simulink library "ddm"  (R2021b)
settings: Solver=VariableStepAuto  StartTime=0.0  StopTime=10.0  RelTol=1e-3
undefined symbols (not defined in the file): ADDM_FrTMTqDev_X_Nm, ADDM_RrTMTqDev_X_Nm, ENUM_ADASACCSTA_ERROR, ENUM_ADASACCSTA_OFF, ENUM_ADASACCSTA_STANDBY, ENUM_ALLOWMOV_ALLOWREADY, ENUM_APS, ENUM_BRKSTA_ERROR, ENUM_BRKSTA_OFF, ENUM_BRKSTA_ON, ENUM_BRKSW_INVALID, ENUM_BRKSW_OFF, ENUM_BRKSW_ON, ENUM_CHGPREACTERRSTA_OBCPRE, ENUM_DCDCFAULTSTA_ANYFAULTLV1, ENUM_DCDCFAULTSTA_ANYFAULTLV2, ENUM_DRIVETRAIN_AWD, ENUM_DRIVETRAIN_FWD, ENUM_DRIVETRAIN_RWD, ENUM_EDUDRTSTA_NORMAL, ENUM_EPBERROR_FAILED, ENUM_EPBSTA_APPLIED, ENUM_EPBSTA_RELEASED, ENUM_ESCAPSSta_APSUNAVAILABLE, ENUM_GEARACTUALPOSN_INVALID, ENUM_GEARACTUALPOSN_P, ENUM_HVBATTREADYPRE_READY, ENUM_HWRESETSTA_HWRESETING, ENUM_MCUWARN_LV0, ENUM_MCUWARN_LV1, ENUM_MCUWARN_LV2, ENUM_MCUWARN_LV3, ENUM_MCUWARN_NOERROR, ENUM_OBCFAULTSTA_ANYFAULT, ENUM_PAS_R2F2, ENUM_PDFAULT_BATTPDFAIL, ENUM_PDFAULT_DCDCDISABLE, ENUM_PDFAULT_MCUDISABLE, ENUM_PDFAULT_MCUDISCHRG, ENUM_POWERSTA_OFF, ENUM_POWERSTA_ON, ENUM_POWERSTA_READY, ENUM_POWERSTA_STANDBY, ENUM_PRESSINDI_LOW, ENUM_PUFAULT_BATTUPFAIL, ENUM_PUFAULT_DCDCENABLEFAIL, ENUM_PUFAULT_PRECHRGCHKFAIL, ENUM_PUFAULT_SAFETYCHKFAIL, ENUM_PWRSTASW_OFF, ENUM_PWRSTASW_OFFA, ENUM_PWRSTASW_OFFCHVCHRG, ENUM_PWRSTASW_OFFCLVCHRG, ENUM_PWRSTASW_ON, ENUM_PWRSTASW_ONHVCHRG, ENUM_PWRSTASW_READY, ENUM_PWRSTASW_STANDBY, ENUM_RAPSErrWarnSta_NORMAL, ENUM_RAPSErrWarnSta_RAPSERRLV1, ENUM_SHIFTCOMMAND_P, ENUM_SHIFTERERRSTA_PBUTTONFAILURE ... (+471)
libraries: hcu_lib x540, simulink x3
(part 17 of 26)

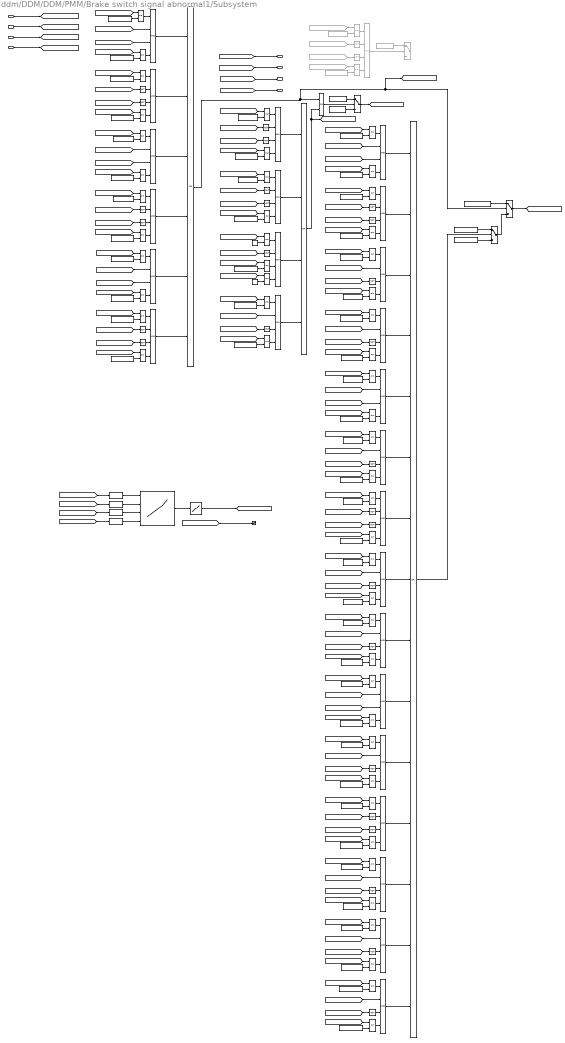
== system ddm/DDM/DDM/PMM/Brake switch signal abnormal1/Subsystem ==
  note: 17
  note: 6
  note: 35
  note: 25
  note: 27
  note: 30
  note: 12
  note: 19
  note: 3
  note: 21
  note: 1
  note: 9
  note: 11
  note: 36
  note: 24
  note: 33
  note: 29
  note: 13
  note: 5
  note: 23
  note: 18
  note: 15
  note: 20
  note: 24
  note: 17
  note: 3
  VDDM_CANBSW2S_enum : Inport
  BrakeSW : Inport  Port=2
  Brake_Stop_Lamp : Inport  Port=3
  BrkPedalPos_enum : Inport  Port=4
  1-D Lookup Table : Lookup_n-D  NumberOfTableDimensions=1  BreakpointsForDimension1=[1:36]  Table=[20,8,32,18,6,30,19,7,31,16,4,28,17,5,29,15,3,27,14,2,26,13,1,25,24,12,36,23,11,35,22,10,34,21,9,33]  ExtrapMethod=Clip  InternalRulePriority=Speed  RndMeth=Simplest  InputSameDT=on
  AND{,2..7,10,12..26,28..29} (25 alike) : Logic  Inputs=4  AllPortsSameDT=off  OutDataTypeStr=boolean
  AND1 : Logic  Operator=OR  Inputs=6  AllPortsSameDT=off  OutDataTypeStr=boolean
  AND11 : Logic  Operator=OR  Inputs=15  AllPortsSameDT=off  OutDataTypeStr=boolean
  AND27 : Logic  Commented=on  Inputs=4  AllPortsSameDT=off  OutDataTypeStr=boolean
  AND8 : Logic  Operator=OR  Inputs=4  AllPortsSameDT=off  OutDataTypeStr=boolean
  AND9 : Logic  Operator=OR  AllPortsSameDT=off  OutDataTypeStr=boolean
  Constant{1..10,15,17..18,23,29..30,32,49,52,54} (20 alike) : Constant  Value=ENUM_BRKSTA_ON
  Constant11 : Constant  Value=ENUM_BRKSW_OFF
  Constant{12..13,20,22,24,33..34,39,41..44,51} (13 alike) : Constant  Value=ENUM_BRKSTA_OFF
  Constant14 : Constant  Commented=on  Value=ENUM_BRKSTA_OFF
  Constant{16,19,21,25..28,31,38,50,53,55,57,59..61} (16 alike) : Constant  Value=ENUM_BRKSTA_ERROR
  Constant35 : Constant  Value=FALSE
  Constant36 : Constant  Value=TRUE
  Constant37 : Constant  Value=0
  Constant40 : Constant  Value=0
  Constant45 : Constant  Commented=on  Value=ENUM_BRKSTA_ERROR
  Constant46 : Constant  Value=ENUM_BRKSW_ON
  Constant47 : Constant  Value=ENUM_BRKSW_INVALID
  Constant48 : Constant  Commented=on  Value=FALSE
  Data Type Conversion{,1..3} (4 alike) : DataTypeConversion
  Equal{1..47,50..53} (51 alike) : RelationalOperator  Operator===  OutDataTypeStr=boolean  RndMeth=Simplest
  Equal48 : RelationalOperator  Commented=on  Operator===  OutDataTypeStr=boolean  RndMeth=Simplest
  Equal49 : RelationalOperator  Commented=on  Operator===  OutDataTypeStr=boolean  RndMeth=Simplest
  From100 : From  Commented=on  GotoTag=BrkPedalPos_enum
  From101 : From  Commented=on  GotoTag=BrakeSW
  From102 : From  Commented=on  GotoTag=VDDM_CANBSW2S_enum
  From103 : From  Commented=on  GotoTag=Brake_Stop_Lamp
  OR{,1..23,26..28} (27 alike) : Logic  Operator=NOT  AllPortsSameDT=off  OutDataTypeStr=boolean
  OR24 : Logic  Commented=on  Operator=NOT  AllPortsSameDT=off  OutDataTypeStr=boolean
  OR25 : Logic  Commented=on  Operator=NOT  AllPortsSameDT=off  OutDataTypeStr=boolean
  Switch1 : Switch  Commented=on  Criteria=u2 > Threshold
  Switch6 : Switch  Criteria=u2 > Threshold
  Switch7 : Switch  Criteria=u2 > Threshold
  Switch8 : Switch  Criteria=u2 > Threshold
  Terminator : Terminator
  n-D Lookup Table : Lookup_n-D  NumberOfTableDimensions=4  BreakpointsForDimension1=[0:2]  BreakpointsForDimension2=[0:1]  BreakpointsForDimension3=[0:1]  BreakpointsForDimension4=[0:2]  Table=reshape(1:36,[3,2,2,3])  ExtrapMethod=Clip  InternalRulePriority=Speed  RndMeth=Simplest  InputSameDT=on
      settings: InputPortMap=u0,u1,u2,u3
  BrkSWErr : Outport
  BrkSWNoBac : Outport  Port=2
  BrkSWPass : Outport  Port=3
  VDDM_BrakeSW_enum : Outport  Port=4
  wires:
  [VDDM_BrakeSigMatrix_enum] -> Terminator/1
  [VDDM_BrakeSW_enum] -> VDDM_BrakeSW_enum/1
  [BrkSWPass] -> BrkSWPass/1
  [BrkSWNoBac] -> BrkSWNoBac/1
  [BrkSWErr] -> BrkSWErr/1
  BrkPedalPos_enum/1 -> [BrkPedalPos_enum]
  Brake_Stop_Lamp/1 -> [Brake_Stop_Lamp]
  BrakeSW/1 -> [BrakeSW]
  VDDM_CANBSW2S_enum/1 -> [VDDM_CANBSW2S_enum]
  AND4/1 -> AND1/4
  Constant28/1 -> Equal14/2
  Constant31/1 -> Equal13/2
  Equal22/1 -> AND10/3
  Constant7/1 -> Equal3/2
  Equal33/1 -> AND19/4
  Equal39/1 -> AND22/4
  OR1/1 -> AND2/3
  [Brake_Stop_Lamp] -> OR8/1
  [Brake_Stop_Lamp] -> OR10/1
  Constant8/1 -> Equal8/2
  Equal17/1 -> AND7/1
  Constant50/1 -> Equal35/2
  Constant32/1 -> Equal41/2
  [BrkPedalPos_enum] -> Equal35/1
  Equal43/1 -> AND24/4
  Constant33/1 -> Equal26/2
  [VDDM_CANBSW2S_enum] -> Equal9/1
  Constant37/1 -> Equal20/2
  [BrkPedalPos_enum] -> Equal45/1
  Switch7/1 -> Switch8/3
  Equal36/1 -> AND21/1
  [Brake_Stop_Lamp] -> AND5/3
  Constant3/1 -> Equal17/2
  Constant44/1 -> Equal43/2
  Constant39/1 -> Equal30/2
  OR8/1 -> AND13/3
  [Brake_Stop_Lamp] -> OR19/1
  [VDDM_CANBSW2S_enum] -> Equal20/1
  Equal20/1 -> AND10/1
  [Brake_Stop_Lamp] -> Equal22/1
  [BrkPedalPos_enum] -> Equal6/1
  [VDDM_CANBSW2S_enum] -> Equal2/1
  Equal5/1 -> AND3/1
  [Brake_Stop_Lamp] -> OR3/1
  [Brake_Stop_Lamp] -> OR15/1
  Constant26/1 -> Equal11/2
  [Brake_Stop_Lamp] -> AND21/3
  OR19/1 -> AND24/3
  [BrkPedalPos_enum] -> Equal10/1
  [BrakeSW] -> AND25/2
  OR3/1 -> AND4/3
  Equal31/1 -> AND18/4
  [BrkPedalPos_enum] -> Equal31/1
  [VDDM_CANBSW2S_enum] -> Equal38/1
  Equal13/1 -> AND6/4
  AND9/1 -> Switch6/2
  [VDDM_CANBSW2S_enum] -> Equal17/1
  [Brake_Stop_Lamp] -> AND16/3
  Equal18/1 -> AND7/4
  [BrkPedalPos_enum] -> Equal27/1
  Constant61/1 -> Equal44/2
  Equal14/1 -> AND6/1
  [VDDM_CANBSW2S_enum] -> Equal5/1
  [VDDM_CANBSW2S_enum] -> Equal28/1
  [VDDM_CANBSW2S_enum] -> Equal3/1
  [BrkPedalPos_enum] -> Equal8/1
  [Brake_Stop_Lamp] -> OR14/1
  Constant30/1 -> Equal16/2
  Constant43/1 -> Equal34/2
  OR13/1 -> AND18/2
  Equal26/1 -> AND16/1
  OR7/1 -> AND13/2
  [BrakeSW] -> AND24/2
  Equal16/1 -> AND/1
  Equal34/1 -> AND20/1
  Equal9/1 -> AND14/1
  Equal12/1 -> AND5/4
  [VDDM_CANBSW2S_enum] -> Equal24/1
  Constant16/1 -> Equal1/2
  Constant18/1 -> Equal31/2
  Constant9/1 -> Equal9/2
  AND2/1 -> AND1/2
  Constant40/1 -> Equal19/2
  OR17/1 -> AND23/2
  AND5/1 -> AND1/5
  AND6/1 -> AND1/6
  Equal37/1 -> AND21/4
  Constant25/1 -> Equal10/2
  [BrkPedalPos_enum] -> Equal15/1
  Constant21/1 -> Equal6/2
  [BrkPedalPos_enum] -> Equal29/1
  [VDDM_CANBSW2S_enum] -> Equal34/1
  [BrkPedalPos_enum] -> Equal23/1
  Constant15/1 -> Equal27/2
  Equal27/1 -> AND16/4
  OR14/1 -> AND19/3
  [BrkPedalPos_enum] -> Equal43/1
  [VDDM_CANBSW2S_enum] -> Equal26/1
  [BrakeSW] -> AND16/2
  Equal24/1 -> AND2/1
  Constant6/1 -> Equal23/2
  OR11/1 -> AND17/3
  [BrakeSW] -> AND14/2
  [BrakeSW] -> AND17/2
  Constant38/1 -> Equal21/2
  [BrkPedalPos_enum] -> Equal41/1
  [BrakeSW] -> AND3/2
  Equal7/1 -> AND4/1
  Equal28/1 -> AND17/1
  OR16/1 -> AND22/3
  Equal23/1 -> AND12/4
  Equal25/1 -> AND15/1
  Constant57/1 -> Equal40/2
  [VDDM_CANBSW2S_enum] -> Equal11/1
  Constant55/1 -> Equal38/2
  OR6/1 -> AND10/2
  Equal10/1 -> AND4/4
  OR9/1 -> AND14/3
  AND8/1 -> [BrkSWPass], AND9/2
  Constant1/1 -> Equal24/2
  [BrakeSW] -> AND20/2
  Equal19/1 -> AND10/4
  Constant36/1 -> Switch6/3
  [VDDM_CANBSW2S_enum] -> Equal40/1
  [BrakeSW] -> AND19/2
  [BrkPedalPos_enum] -> Equal1/1
  Constant4/1 -> Equal18/2
  [VDDM_CANBSW2S_enum] -> Equal14/1
  [Brake_Stop_Lamp] -> AND/3
  [BrkPedalPos_enum] -> Equal37/1
  Constant60/1 -> Equal45/2
  Constant5/1 -> Equal2/2
  Constant20/1 -> Equal5/2
  [BrakeSW] -> AND22/2
  [BrakeSW] -> AND21/2
  Constant53/1 -> Equal36/2
  Equal35/1 -> AND20/4
  [VDDM_CANBSW2S_enum] -> Equal16/1
  [BrakeSW] -> OR7/1
  Constant10/1 -> Equal25/2
  [Brake_Stop_Lamp] -> OR5/1
  [Brake_Stop_Lamp] -> AND3/3
  Equal6/1 -> AND3/4
  Constant42/1 -> Equal33/2
  [VDDM_CANBSW2S_enum] -> Equal30/1
  [BrakeSW] -> OR/1
  Equal41/1 -> AND23/4
  OR12/1 -> AND18/3
  [Brake_Stop_Lamp] -> OR12/1
  [VDDM_CANBSW2S_enum] -> Equal36/1
  Constant24/1 -> Equal15/2
  [Brake_Stop_Lamp] -> OR16/1
  Constant41/1 -> Equal32/2
  Equal32/1 -> AND19/1
  Switch8/1 -> [VDDM_BrakeSW_enum]
  Constant17/1 -> Equal29/2
  Equal45/1 -> AND25/4
  Constant19/1 -> Equal4/2
  [BrakeSW] -> AND7/2
  OR21/1 -> AND7/3
  Constant47/1 -> Switch8/1
  [Brake_Stop_Lamp] -> OR21/1
  [Brake_Stop_Lamp] -> OR9/1
  Equal40/1 -> AND23/1
  Equal3/1 -> AND13/1
  Equal11/1 -> AND5/1
  Equal38/1 -> AND22/1
  Constant11/1 -> Switch7/3
  Equal1/1 -> AND/4
  Switch6/1 -> [BrkSWErr]
  [BrkPedalPos_enum] -> Equal13/1
  [BrkPedalPos_enum] -> Equal21/1
  Constant35/1 -> Switch6/1
  AND/1 -> AND1/1
  Constant34/1 -> Equal28/2
  [VDDM_CANBSW2S_enum] -> Equal44/1
  OR10/1 -> AND15/3
  [Brake_Stop_Lamp] -> AND12/3
  [BrkPedalPos_enum] -> Equal18/1
  Equal8/1 -> AND13/4
  Equal2/1 -> AND12/1
  [BrkPedalPos_enum] -> Equal4/1
  [Brake_Stop_Lamp] -> OR11/1
  Equal44/1 -> AND25/1
  Equal42/1 -> AND24/1
  [BrakeSW] -> OR4/1
  OR20/1 -> AND25/3
  [VDDM_CANBSW2S_enum] -> Equal7/1
  OR4/1 -> AND6/2
  Constant23/1 -> Equal37/2
  [VDDM_CANBSW2S_enum] -> Equal32/1
  [VDDM_CANBSW2S_enum] -> Equal42/1
  [BrkPedalPos_enum] -> Equal19/1
  [BrkPedalPos_enum] -> Equal12/1
  [BrkPedalPos_enum] -> Equal39/1
  [BrakeSW] -> OR6/1
  Constant59/1 -> Equal42/2
  AND1/1 -> Switch8/2, [BrkSWNoBac], AND9/1
  Constant27/1 -> Equal12/2
  [BrakeSW] -> AND15/2
  Constant46/1 -> Switch7/1
  AND11/1 -> Switch7/2
  [BrakeSW] -> OR2/1
  [VDDM_CANBSW2S_enum] -> Equal25/1
  Constant2/1 -> Equal22/2
  [Brake_Stop_Lamp] -> OR1/1
  [Brake_Stop_Lamp] -> OR18/1
  [BrakeSW] -> OR13/1
  OR5/1 -> AND6/3
  Constant22/1 -> Equal7/2
  Constant29/1 -> Equal39/2
  OR18/1 -> AND23/3
  [BrakeSW] -> AND/2
  [BrakeSW] -> OR17/1
  AND3/1 -> AND1/3
  [BrakeSW] -> AND12/2
  [Brake_Stop_Lamp] -> OR20/1
  OR15/1 -> AND20/3
  OR/1 -> AND2/2
  Equal21/1 -> AND15/4
  Equal30/1 -> AND18/1
  Equal29/1 -> AND17/4
  Equal15/1 -> AND14/4
  [BrakeSW] -> AND5/2
  OR2/1 -> AND4/2
  Equal4/1 -> AND2/4
  [BrkPedalPos_enum] -> Equal33/1
  Data Type Conversion2/1 -> n-D Lookup Table/3
  Data Type Conversion3/1 -> n-D Lookup Table/4
  Data Type Conversion1/1 -> n-D Lookup Table/2
  Data Type Conversion/1 -> n-D Lookup Table/1
  [BrakeSW] -> Data Type Conversion1/1
  [BrkPedalPos_enum] -> Data Type Conversion3/1
  n-D Lookup Table/1 -> 1-D Lookup Table/1
  [Brake_Stop_Lamp] -> Data Type Conversion2/1
  1-D Lookup Table/1 -> [VDDM_BrakeSigMatrix_enum]  "VDDM_BrakeSigMatrix_enum"
  [VDDM_CANBSW2S_enum] -> Data Type Conversion/1
  [BrkPedalPos_enum] -> Equal47/1
  OR22/1 -> AND26/2
  OR23/1 -> AND26/3
  [BrakeSW] -> OR22/1
  Constant13/1 -> Equal47/2
  Equal47/1 -> AND26/4
  [Brake_Stop_Lamp] -> OR23/1
  [VDDM_CANBSW2S_enum] -> Equal46/1
  Constant12/1 -> Equal46/2
  Equal46/1 -> AND26/1
  AND27/1 -> Switch1/2
  Equal49/1 -> AND27/1
  From102/1 -> Equal49/1
  OR25/1 -> AND27/3
  Constant14/1 -> Equal49/2
  From101/1 -> OR24/1
  OR24/1 -> AND27/2
  From103/1 -> OR25/1
  Equal48/1 -> AND27/4
  Constant45/1 -> Equal48/2
  From100/1 -> Equal48/1
  Constant48/1 -> Switch1/1
  Constant49/1 -> Equal51/2
  OR27/1 -> AND28/2
  Equal51/1 -> AND28/4
  [Brake_Stop_Lamp] -> OR26/1
  Constant51/1 -> Equal50/2
  Equal50/1 -> AND28/1
  [BrakeSW] -> OR27/1
  [BrkPedalPos_enum] -> Equal51/1
  [VDDM_CANBSW2S_enum] -> Equal50/1
  OR26/1 -> AND28/3
  AND26/1 -> AND8/1
  AND28/1 -> AND8/2
  AND10/1 -> AND8/3
  AND7/1 -> AND8/4
  AND12/1 -> AND11/1
  AND13/1 -> AND11/2
  AND14/1 -> AND11/3
  AND15/1 -> AND11/4
  AND16/1 -> AND11/5
  AND25/1 -> AND11/14
  AND24/1 -> AND11/13
  AND23/1 -> AND11/12
  AND22/1 -> AND11/11
  AND21/1 -> AND11/10
  AND20/1 -> AND11/9
  AND19/1 -> AND11/8
  AND18/1 -> AND11/7
  AND17/1 -> AND11/6
  Constant52/1 -> Equal52/2
  Equal52/1 -> AND29/1
  [BrakeSW] -> AND29/2
  Equal53/1 -> AND29/4
  [Brake_Stop_Lamp] -> OR28/1
  [VDDM_CANBSW2S_enum] -> Equal52/1
  [BrkPedalPos_enum] -> Equal53/1
  AND29/1 -> AND11/15
  OR28/1 -> AND29/3
  Constant54/1 -> Equal53/2

== system ddm/DDM/DDM/PMM/Comm err/The CAN signal between VCU and ABM1 is discontinuous ==
  note: Diagnostics and Fault Handling
  note: Test Pass Criteria
  note: Release Condition After Decision
  note: Test Detection Criteria
  task_time_s : Inport
  VPMM_PowerSta_enum : Inport  Port=2
  VPMM_PwrStaSW_enum : Inport  Port=3
  VDDM_C1ABM1RCChk_flg : Inport  Port=4
  VDDM_C1ABM1LCCFS_flg : Inport  Port=5
  No_CAN1_BUS_OFF : Inport  Port=6
  DTC_clear_request : Inport  Port=7
  Constant1 : Constant  Value=TRUE
  Constant10 : Constant  Value=ENUM_POWERSTA_STANDBY
  Constant11 : Constant  Value=ZERO_INT
  Constant12 : Constant  Value=FALSE
  Constant13 : Constant  Value=KDDM_C1ABM1RCDetTO_s
  Constant14 : Constant  Value=KDDM_C1ABM1RCPassTO_s
  Constant17 : Constant  Value=KDDM_C1ABM1RCPassTO_s
  Constant29 : Constant  Value=ENUM_PWRSTASW_OFF
  Constant30 : Constant  Value=KDDM_CommErrDiagnosisOffSW_flg
  Constant31 : Constant  Value=ENUM_POWERSTA_OFF
  Constant6 : Constant  Value=KDDM_C1ABM1RCDTC_cnt
  Constant7 : Constant  Value=KDDM_C1ABM1RCDTC_cnt
  Constant8 : Constant  Value=FALSE
  Constant9 : Constant  Value=ENUM_PWRSTASW_OFF
  DTC_Couter1 : hcu_lib/Basic_Blocks/DTC_Couter
  DTC_Info : hcu_lib/Basic_Blocks/DTC_Info
  Equal1 : RelationalOperator  Operator=~=  OutDataTypeStr=boolean  RndMeth=Simplest
  Equal5 : RelationalOperator  Operator=~=  OutDataTypeStr=boolean  RndMeth=Simplest
  Equal6 : RelationalOperator  OutDataTypeStr=boolean  RndMeth=Simplest
  Equal7 : RelationalOperator  Operator===  OutDataTypeStr=boolean  RndMeth=Simplest
  Equal8 : RelationalOperator  Operator===  OutDataTypeStr=boolean  RndMeth=Simplest
  Logical Operator11 : Logic  Operator=NOT  AllPortsSameDT=off  OutDataTypeStr=boolean
  Logical Operator13 : Logic  Inputs=3  AllPortsSameDT=off  OutDataTypeStr=boolean
  Logical Operator14 : Logic  Operator=NOT  AllPortsSameDT=off  OutDataTypeStr=boolean
  Logical Operator16 : Logic  Operator=OR  Inputs=4  AllPortsSameDT=off  OutDataTypeStr=boolean
  Logical Operator17 : Logic  AllPortsSameDT=off  OutDataTypeStr=boolean
  Logical Operator20 : Logic  Inputs=3  AllPortsSameDT=off  OutDataTypeStr=boolean
  Logical Operator21 : Logic  Operator=NOT  AllPortsSameDT=off  OutDataTypeStr=boolean
  Relational Operator1 : RelationalOperator  Operator=>  OutDataTypeStr=boolean  RndMeth=Simplest
  Switch2 : Switch  Criteria=u2 ~= 0
  Switch8 : Switch  Criteria=u2 ~= 0
  Switch9 : Switch  Criteria=u2 ~= 0
  Terminator : Terminator
  Test Detection Criteria1 : hcu_lib/Basic_Blocks/Test Detection Criteria
  Timer2 : hcu_lib/Basic_Blocks/Timer
  Unit Delay1 : UnitDelay  SampleTime=-1  HasFrameUpgradeWarning=on
  VDDM_C1ABM1RCDTC_raw32 : Outport
  RC_EDriveSysErr_VCUErr_flg : Outport  Port=2
  VDDM_C1ABM1RCCFS_flg : Outport  Port=3
  wires:
  [DTC_clear_request] -> DTC_Info/4
  [VDDM_C1ABM1RCDet_flg] -> DTC_Info/1
  [VDDM_C1ABM1RCCFS_flg] -> DTC_Info/3
  [VDDM_C1ABM1RCPass_flg] -> DTC_Info/2
  DTC_Info/1 -> VDDM_C1ABM1RCDTC_raw32/1  "VDDM_C1ABM1RCDTC_raw32"
  [VDDM_C1ABM1RCCFS_flg] -> RC_EDriveSysErr_VCUErr_flg/1, VDDM_C1ABM1RCCFS_flg/1
  DTC_clear_request/1 -> [DTC_clear_request]
  No_CAN1_BUS_OFF/1 -> [No_CAN1_BUS_OFF]
  VDDM_C1ABM1LCCFS_flg/1 -> [VDDM_C1ABM1LCCFS_flg]
  VPMM_PowerSta_enum/1 -> [VPMM_PowerSta_enum]
  VPMM_PwrStaSW_enum/1 -> [VPMM_PwrStaSW_enum]
  VDDM_C1ABM1RCChk_flg/1 -> [VDDM_C1ABM1RCChk_flg]
  task_time_s/1 -> [task_time_s]
  [VDDM_C1ABM1LCCFS_flg] -> Logical Operator11/1
  [VDDM_C1ABM1RCCFSRls_flg] -> DTC_Couter1/2
  Constant8/1 -> Switch9/1
  Timer2/1 -> Equal6/1
  Equal1/1 -> Logical Operator13/2
  Constant12/1 -> Switch2/3
  Constant17/1 -> Equal6/2
  Equal8/1 -> Logical Operator17/2
  Logical Operator21/1 -> Timer2/1
  DTC_Couter1/2 -> Relational Operator1/1  "VDDM_C1ABM1RCDTC_cnt"
  Constant31/1 -> Equal7/2
  [No_CAN1_BUS_OFF] -> Logical Operator20/1
  Logical Operator17/1 -> Logical Operator16/1
  [task_time_s] -> Timer2/3
  Constant9/1 -> Equal1/2
  [VPMM_PowerSta_enum] -> Equal8/1
  Switch9/1 -> Test Detection Criteria1/1
  [VDDM_C1ABM1RCPass_flg] -> Logical Operator16/3
  Constant10/1 -> Equal8/2
  Constant30/1 -> Logical Operator16/4
  Constant1/1 -> Switch8/3
  Switch2/1 -> Switch9/3
  [DTC_clear_request] -> Logical Operator16/2
  [VDDM_C1ABM1RCChk_flg] -> Switch8/1
  [VPMM_PowerSta_enum] -> Unit Delay1/1
  Equal5/1 -> Logical Operator20/2
  [No_CAN1_BUS_OFF] -> Logical Operator13/1
  [task_time_s] -> Test Detection Criteria1/2
  [VPMM_PwrStaSW_enum] -> Equal1/1
  Relational Operator1/1 -> Terminator/1  "VDDM_C1ABM1RCDFS_flg"
  [VPMM_PwrStaSW_enum] -> Equal5/1
  Equal7/1 -> Logical Operator17/1
  [VDDM_C1ABM1RCDet_flg] -> DTC_Couter1/1
  Logical Operator13/1 -> Switch2/2
  [VDDM_C1ABM1RCChk_flg] -> Switch2/1
  Switch8/1 -> Timer2/2, Logical Operator21/1
  [VDDM_C1ABM1LCCFS_flg] -> Logical Operator14/1
  DTC_Couter1/1 -> [VDDM_C1ABM1RCCFS_flg]  "VDDM_C1ABM1RCCFS_flg"
  Constant6/1 -> Test Detection Criteria1/3
  Equal6/1 -> [VDDM_C1ABM1RCPass_flg]  "VDDM_C1ABM1RCPass_flg"
  Constant7/1 -> DTC_Couter1/3
  Constant14/1 -> Timer2/4
  Test Detection Criteria1/1 -> [VDDM_C1ABM1RCDet_flg]  "VDDM_C1ABM1RCDet_flg"
  Constant11/1 -> Relational Operator1/2
  Constant13/1 -> Test Detection Criteria1/4
  Logical Operator16/1 -> [VDDM_C1ABM1RCCFSRls_flg]  "VDDM_C1ABM1RCCFSRls_flg"
  Logical Operator11/1 -> Logical Operator13/3
  Constant29/1 -> Equal5/2
  Unit Delay1/1 -> Equal7/1
  Logical Operator14/1 -> Logical Operator20/3
  [VDDM_C1ABM1RCCFSRls_flg] -> Switch9/2
  Logical Operator20/1 -> Switch8/2

== system ddm/DDM/DDM/PMM/Comm err/The CAN signal between VCU and ABM1 is incomplete ==
  note: Test Pass Criteria
  note: Diagnostics and Fault Handling
  note: Test Detection Criteria
  note: Release Condition After Decision
  task_time_s : Inport
  VPMM_PowerSta_enum : Inport  Port=2
  VPMM_PwrStaSW_enum : Inport  Port=3
  VDDM_C1ABM1CSChk_flg : Inport  Port=4
  VDDM_C1ABM1LCCFS_flg : Inport  Port=5
  No_CAN1_BUS_OFF : Inport  Port=6
  DTC_clear_request : Inport  Port=7
  Constant1 : Constant  Value=KDDM_C1ABM1CSDTC_cnt
  Constant10 : Constant  Value=ENUM_POWERSTA_STANDBY
  Constant11 : Constant  Value=ZERO_INT
  Constant12 : Constant  Value=ENUM_PWRSTASW_OFF
  Constant13 : Constant  Value=FALSE
  Constant14 : Constant  Value=KDDM_C1ABM1CSPassTO_s
  Constant17 : Constant  Value=KDDM_C1ABM1CSPassTO_s
  Constant29 : Constant  Value=ENUM_PWRSTASW_OFF
  Constant30 : Constant  Value=KDDM_CommErrDiagnosisOffSW_flg
  Constant31 : Constant  Value=ENUM_POWERSTA_OFF
  Constant6 : Constant  Value=TRUE
  Constant7 : Constant  Value=KDDM_C1ABM1CSDTC_cnt
  Constant8 : Constant  Value=KDDM_C1ABM1CSDetTO_s
  Constant9 : Constant  Value=FALSE
  DTC_Couter1 : hcu_lib/Basic_Blocks/DTC_Couter
  DTC_Info : hcu_lib/Basic_Blocks/DTC_Info
  Equal1 : RelationalOperator  Operator=~=  OutDataTypeStr=boolean  RndMeth=Simplest
  Equal5 : RelationalOperator  Operator=~=  OutDataTypeStr=boolean  RndMeth=Simplest
  Equal6 : RelationalOperator  OutDataTypeStr=boolean  RndMeth=Simplest
  Equal7 : RelationalOperator  Operator===  OutDataTypeStr=boolean  RndMeth=Simplest
  Equal8 : RelationalOperator  Operator===  OutDataTypeStr=boolean  RndMeth=Simplest
  Logical Operator11 : Logic  Operator=NOT  AllPortsSameDT=off  OutDataTypeStr=boolean
  Logical Operator13 : Logic  Inputs=3  AllPortsSameDT=off  OutDataTypeStr=boolean
  Logical Operator14 : Logic  Operator=NOT  AllPortsSameDT=off  OutDataTypeStr=boolean
  Logical Operator16 : Logic  Operator=OR  Inputs=4  AllPortsSameDT=off  OutDataTypeStr=boolean
  Logical Operator17 : Logic  AllPortsSameDT=off  OutDataTypeStr=boolean
  Logical Operator20 : Logic  Inputs=3  AllPortsSameDT=off  OutDataTypeStr=boolean
  Logical Operator21 : Logic  Operator=NOT  AllPortsSameDT=off  OutDataTypeStr=boolean
  Relational Operator1 : RelationalOperator  Operator=>  OutDataTypeStr=boolean  RndMeth=Simplest
  Switch2 : Switch  Criteria=u2 ~= 0
  Switch8 : Switch  Criteria=u2 ~= 0
  Switch9 : Switch  Criteria=u2 ~= 0
  Terminator : Terminator
  Test Detection Criteria1 : hcu_lib/Basic_Blocks/Test Detection Criteria
  Timer2 : hcu_lib/Basic_Blocks/Timer
  Unit Delay1 : UnitDelay  SampleTime=-1  HasFrameUpgradeWarning=on
  VDDM_C1ABM1CSDTC_raw32 : Outport
  CS_EDriveSysErr_VCUErr_flg : Outport  Port=2
  VDDM_C1ABM1CSCFS_flg : Outport  Port=3
  wires:
  [DTC_clear_request] -> DTC_Info/4
  [VDDM_C1ABM1CSDet_flg] -> DTC_Info/1
  [VDDM_C1ABM1CSPass_flg] -> DTC_Info/2
  [VDDM_C1ABM1CSCFS_flg] -> DTC_Info/3
  DTC_Info/1 -> VDDM_C1ABM1CSDTC_raw32/1  "VDDM_C1ABM1CSDTC_raw32"
  [VDDM_C1ABM1CSCFS_flg] -> CS_EDriveSysErr_VCUErr_flg/1, VDDM_C1ABM1CSCFS_flg/1
  No_CAN1_BUS_OFF/1 -> [No_CAN1_BUS_OFF]
  DTC_clear_request/1 -> [DTC_clear_request]
  task_time_s/1 -> [task_time_s]
  VDDM_C1ABM1CSChk_flg/1 -> [VDDM_C1ABM1CSChk_flg]
  VPMM_PwrStaSW_enum/1 -> [VPMM_PwrStaSW_enum]
  VPMM_PowerSta_enum/1 -> [VPMM_PowerSta_enum]
  VDDM_C1ABM1LCCFS_flg/1 -> [VDDM_C1ABM1LCCFS_flg]
  [DTC_clear_request] -> Logical Operator16/2
  Constant13/1 -> Switch2/3
  Constant7/1 -> Test Detection Criteria1/3
  Constant17/1 -> Equal6/2
  [No_CAN1_BUS_OFF] -> Logical Operator13/1
  Constant8/1 -> Test Detection Criteria1/4
  Logical Operator13/1 -> Switch2/2
  Constant14/1 -> Timer2/4
  Constant12/1 -> Equal1/2
  Relational Operator1/1 -> Terminator/1  "VDDM_C1ABM1CSDFS_flg"
  Constant10/1 -> Equal8/2
  Constant9/1 -> Switch9/1
  Equal6/1 -> [VDDM_C1ABM1CSPass_flg]  "VDDM_C1ABM1CSPass_flg"
  [task_time_s] -> Test Detection Criteria1/2
  Equal5/1 -> Logical Operator20/2
  [VPMM_PowerSta_enum] -> Equal8/1
  [VDDM_C1ABM1CSChk_flg] -> Switch2/1
  Equal8/1 -> Logical Operator17/2
  [VDDM_C1ABM1CSDet_flg] -> DTC_Couter1/1
  [VPMM_PwrStaSW_enum] -> Equal5/1
  [VPMM_PowerSta_enum] -> Unit Delay1/1
  Test Detection Criteria1/1 -> [VDDM_C1ABM1CSDet_flg]  "VDDM_C1ABM1CSDet_flg"
  Logical Operator14/1 -> Logical Operator20/3
  Constant11/1 -> Relational Operator1/2
  [VDDM_C1ABM1CSPass_flg] -> Logical Operator16/3
  Timer2/1 -> Equal6/1
  Constant1/1 -> DTC_Couter1/3
  Logical Operator17/1 -> Logical Operator16/1
  Constant29/1 -> Equal5/2
  Constant6/1 -> Switch8/3
  Equal1/1 -> Logical Operator13/2
  Switch9/1 -> Test Detection Criteria1/1
  Switch8/1 -> Timer2/2, Logical Operator21/1
  Constant31/1 -> Equal7/2
  [No_CAN1_BUS_OFF] -> Logical Operator20/1
  Switch2/1 -> Switch9/3
  Equal7/1 -> Logical Operator17/1
  [task_time_s] -> Timer2/3
  Logical Operator20/1 -> Switch8/2
  [VDDM_C1ABM1CSChk_flg] -> Switch8/1
  DTC_Couter1/2 -> Relational Operator1/1  "VDDM_C1ABM1CSDTC_cnt"
  DTC_Couter1/1 -> [VDDM_C1ABM1CSCFS_flg]  "VDDM_C1ABM1CSCFS_flg"
  Logical Operator21/1 -> Timer2/1
  [VDDM_C1ABM1CSCFSRls_flg] -> DTC_Couter1/2
  [VDDM_C1ABM1LCCFS_flg] -> Logical Operator14/1
  Logical Operator11/1 -> Logical Operator13/3
  Unit Delay1/1 -> Equal7/1
  [VPMM_PwrStaSW_enum] -> Equal1/1
  [VDDM_C1ABM1LCCFS_flg] -> Logical Operator11/1
  Constant30/1 -> Logical Operator16/4
  [VDDM_C1ABM1CSCFSRls_flg] -> Switch9/2
  Logical Operator16/1 -> [VDDM_C1ABM1CSCFSRls_flg]  "VDDM_C1ABM1CSCFSRls_flg"

== system ddm/DDM/DDM/PMM/Comm err/The CAN signal between VCU and BMS1 is discontinuous ==
  note: Test Detection Criteria
  note: Test Pass Criteria
  note: Release Condition After Decision
  note: Diagnostics and Fault Handling
  task_time_s : Inport
  VPMM_PowerSta_enum : Inport  Port=2
  VPMM_PwrStaSW_enum : Inport  Port=3
  VDDM_C3BMS1RCChk_flg : Inport  Port=4
  VDDM_C3BMS1LCCFS_flg : Inport  Port=5
  No_CAN3_BUS_OFF : Inport  Port=6
  DTC_clear_request : Inport  Port=7
  VPMM_HWResetSta_enum : Inport  Port=8
  Constant1 : Constant  Value=TRUE
  Constant10 : Constant  Value=ENUM_POWERSTA_STANDBY
  Constant11 : Constant  Value=ZERO_INT
  Constant12 : Constant  Value=FALSE
  Constant13 : Constant  Value=KDDM_C3BMS1RCDTC_cnt
  Constant14 : Constant  Value=KDDM_C3BMS1RCDetTO_s
  Constant17 : Constant  Value=KDDM_C3BMS1RCDTC_cnt
  Constant2 : Constant  Value=ENUM_HWRESETSTA_HWRESETING
  Constant3 : Constant  Value=ENUM_PWRSTASW_OFF
  Constant30 : Constant  Value=KDDM_CommErrDiagnosisOffSW_flg
  Constant31 : Constant  Value=ENUM_POWERSTA_OFF
  Constant5 : Constant  Value=ENUM_HWRESETSTA_HWRESETING
  Constant6 : Constant  Value=KDDM_C3BMS1RCPassTO_s
  Constant7 : Constant  Value=KDDM_C3BMS1RCPassTO_s
  Constant8 : Constant  Value=FALSE
  Constant9 : Constant  Value=ENUM_PWRSTASW_OFF
  DTC_Couter1 : hcu_lib/Basic_Blocks/DTC_Couter
  DTC_Info : hcu_lib/Basic_Blocks/DTC_Info
  Delay1 : Delay  DelayLength=1
  Equal{1..4} (4 alike) : RelationalOperator  Operator=~=  OutDataTypeStr=boolean  RndMeth=Simplest
  Equal6 : RelationalOperator  OutDataTypeStr=boolean  RndMeth=Simplest
  Equal7 : RelationalOperator  Operator===  OutDataTypeStr=boolean  RndMeth=Simplest
  Equal8 : RelationalOperator  Operator===  OutDataTypeStr=boolean  RndMeth=Simplest
  Logical Operator1 : Logic  Operator=NOT  AllPortsSameDT=off  OutDataTypeStr=boolean
  Logical Operator10 : Logic  Operator=NOT  AllPortsSameDT=off  OutDataTypeStr=boolean
  Logical Operator11 : Logic  Inputs=4  AllPortsSameDT=off  OutDataTypeStr=boolean
  Logical Operator14 : Logic  Operator=OR  Inputs=4  AllPortsSameDT=off  OutDataTypeStr=boolean
  Logical Operator16 : Logic  AllPortsSameDT=off  OutDataTypeStr=boolean
  Logical Operator2 : Logic  Inputs=4  AllPortsSameDT=off  OutDataTypeStr=boolean
  Logical Operator20 : Logic  Operator=NOT  AllPortsSameDT=off  OutDataTypeStr=boolean
  Logical Operator22 : Logic  AllPortsSameDT=off  OutDataTypeStr=boolean
  NOT1 : Logic  Operator=NOT  AllPortsSameDT=off  OutDataTypeStr=boolean
  Relational Operator1 : RelationalOperator  Operator=>  OutDataTypeStr=boolean  RndMeth=Simplest
  Switch1 : Switch  Criteria=u2 ~= 0
  Switch2 : Switch  Criteria=u2 ~= 0
  Switch9 : Switch  Criteria=u2 ~= 0
  Terminator : Terminator
  Test Detection Criteria : hcu_lib/Basic_Blocks/Test Detection Criteria
  Timer2 : hcu_lib/Basic_Blocks/Timer
  Unit Delay1 : UnitDelay  SampleTime=-1  HasFrameUpgradeWarning=on
  VDDM_C3BMS1RCDTC_raw32 : Outport
  VDDM_C3BMS1RCCFS_flg : Outport  Port=2
  wires:
  Constant3/1 -> Equal3/2
  [No_CAN3_BUS_OFF] -> Logical Operator2/1
  Constant1/1 -> Switch1/3
  [VDDM_C3BMS1LCCFS_flg] -> Logical Operator1/1
  Equal4/1 -> Logical Operator2/4
  Logical Operator2/1 -> Switch1/2
  Logical Operator1/1 -> Logical Operator2/3
  [VDDM_C3BMS1RCChk_flg] -> Switch1/1
  [VPMM_PwrStaSW_enum] -> Equal3/1
  Equal3/1 -> Logical Operator2/2
  [VPMM_HWResetSta_enum] -> Equal4/1
  Constant2/1 -> Equal4/2
  Equal2/1 -> Logical Operator11/4
  Constant5/1 -> Equal2/2
  [VPMM_HWResetSta_enum] -> Equal2/1
  VPMM_HWResetSta_enum/1 -> [VPMM_HWResetSta_enum]
  [VDDM_C3BMS1RCCFS_flg] -> VDDM_C3BMS1RCCFS_flg/1
  DTC_Couter1/2 -> Relational Operator1/1  "VDDM_C3BMS1RCDTC_cnt"
  Constant6/1 -> Timer2/4
  DTC_Couter1/1 -> [VDDM_C3BMS1RCCFS_flg]  "VDDM_C3BMS1RCCFS_flg"
  Delay1/1 -> NOT1/1
  [VDDM_C3BMS1RCDet_flg] -> DTC_Couter1/1
  Logical Operator16/1 -> Logical Operator14/1
  Unit Delay1/1 -> Equal7/1
  Equal1/1 -> Logical Operator11/2
  [DTC_clear_request] -> Logical Operator14/2
  Constant31/1 -> Equal7/2
  Equal7/1 -> Logical Operator16/1
  Test Detection Criteria/1 -> [VDDM_C3BMS1RCDet_flg]  "VDDM_C3BMS1RCDet_flg"
  [VPMM_PowerSta_enum] -> Equal8/1
  Switch9/1 -> Test Detection Criteria/1
  Constant30/1 -> Logical Operator14/4
  Constant10/1 -> Equal8/2
  [task_time_s] -> Timer2/3
  Logical Operator14/1 -> [VDDM_C3BMS1RCCFSRls_flg]  "VDDM_C3BMS1RCCFSRls_flg"
  [VDDM_C3BMS1RCCFS_flg] -> Delay1/1
  Constant13/1 -> Test Detection Criteria/3
  [VPMM_PowerSta_enum] -> Unit Delay1/1
  Relational Operator1/1 -> Terminator/1  "VDDM_C3BMS1RCDFS_flg"
  NOT1/1 -> Logical Operator22/2
  Logical Operator22/1 -> Logical Operator14/3
  Equal8/1 -> Logical Operator16/2
  Constant9/1 -> Equal1/2
  [VDDM_C3BMS1RCPass_flg] -> Logical Operator22/1
  [task_time_s] -> Test Detection Criteria/2
  Switch2/1 -> Switch9/3
  Logical Operator11/1 -> Switch2/2
  [No_CAN3_BUS_OFF] -> Logical Operator11/1
  Constant17/1 -> DTC_Couter1/3
  [VDDM_C3BMS1RCChk_flg] -> Switch2/1
  Equal6/1 -> [VDDM_C3BMS1RCPass_flg]  "VDDM_C3BMS1RCPass_flg"
  [VDDM_C3BMS1RCCFSRls_flg] -> Switch9/2
  [VPMM_PwrStaSW_enum] -> Equal1/1
  Constant8/1 -> Switch9/1
  Constant14/1 -> Test Detection Criteria/4
  Logical Operator10/1 -> Logical Operator11/3
  Constant7/1 -> Equal6/2
  [VDDM_C3BMS1LCCFS_flg] -> Logical Operator10/1
  Switch1/1 -> Logical Operator20/1, Timer2/2
  Timer2/1 -> Equal6/1
  Constant12/1 -> Switch2/3
  Logical Operator20/1 -> Timer2/1
  [VDDM_C3BMS1RCCFSRls_flg] -> DTC_Couter1/2
  Constant11/1 -> Relational Operator1/2
  VPMM_PowerSta_enum/1 -> [VPMM_PowerSta_enum]
  VPMM_PwrStaSW_enum/1 -> [VPMM_PwrStaSW_enum]
  VDDM_C3BMS1RCChk_flg/1 -> [VDDM_C3BMS1RCChk_flg]
  task_time_s/1 -> [task_time_s]
  VDDM_C3BMS1LCCFS_flg/1 -> [VDDM_C3BMS1LCCFS_flg]
  No_CAN3_BUS_OFF/1 -> [No_CAN3_BUS_OFF]
  DTC_clear_request/1 -> [DTC_clear_request]
  [VDDM_C3BMS1RCPass_flg] -> DTC_Info/2
  [VDDM_C3BMS1RCCFS_flg] -> DTC_Info/3
  DTC_Info/1 -> VDDM_C3BMS1RCDTC_raw32/1  "VDDM_C3BMS1RCDTC_raw32"
  [VDDM_C3BMS1RCDet_flg] -> DTC_Info/1
  [DTC_clear_request] -> DTC_Info/4

== system ddm/DDM/DDM/PMM/Comm err/The CAN signal between VCU and BMS1 is incomplete ==
  note: Test Detection Criteria
  note: Release Condition After Decision
  note: Diagnostics and Fault Handling
  note: Test Pass Criteria
  task_time_s : Inport
  VPMM_PowerSta_enum : Inport  Port=2
  VPMM_PwrStaSW_enum : Inport  Port=3
  VDDM_C3BMS1CSChk_flg : Inport  Port=4
  VDDM_C3BMS1LCCFS_flg : Inport  Port=5
  No_CAN3_BUS_OFF : Inport  Port=6
  DTC_clear_request : Inport  Port=7
  VPMM_HWResetSta_enum : Inport  Port=8
  Constant1 : Constant  Value=KDDM_C3BMS1CSDTC_cnt
  Constant10 : Constant  Value=ENUM_POWERSTA_STANDBY
  Constant11 : Constant  Value=ZERO_INT
  Constant12 : Constant  Value=ENUM_PWRSTASW_OFF
  Constant13 : Constant  Value=FALSE
  Constant14 : Constant  Value=KDDM_C3BMS1CSPassTO_s
  Constant2 : Constant  Value=ENUM_HWRESETSTA_HWRESETING
  Constant3 : Constant  Value=ENUM_PWRSTASW_OFF
  Constant30 : Constant  Value=KDDM_CommErrDiagnosisOffSW_flg
  Constant31 : Constant  Value=ENUM_POWERSTA_OFF
  Constant32 : Constant  Value=KDDM_C3BMS1CSDTC_cnt
  Constant33 : Constant  Value=KDDM_C3BMS1CSDetTO_s
  Constant4 : Constant  Value=TRUE
  Constant5 : Constant  Value=ENUM_HWRESETSTA_HWRESETING
  Constant7 : Constant  Value=KDDM_C3BMS1CSPassTO_s
  Constant9 : Constant  Value=FALSE
  DTC_Couter1 : hcu_lib/Basic_Blocks/DTC_Couter
  DTC_Info : hcu_lib/Basic_Blocks/DTC_Info
  Delay1 : Delay  DelayLength=1
  Equal{1..4} (4 alike) : RelationalOperator  Operator=~=  OutDataTypeStr=boolean  RndMeth=Simplest
  Equal6 : RelationalOperator  OutDataTypeStr=boolean  RndMeth=Simplest
  Equal7 : RelationalOperator  Operator===  OutDataTypeStr=boolean  RndMeth=Simplest
  Equal8 : RelationalOperator  Operator===  OutDataTypeStr=boolean  RndMeth=Simplest
  Logical Operator1 : Logic  Operator=NOT  AllPortsSameDT=off  OutDataTypeStr=boolean
  Logical Operator10 : Logic  Operator=NOT  AllPortsSameDT=off  OutDataTypeStr=boolean
  Logical Operator14 : Logic  Operator=OR  Inputs=4  AllPortsSameDT=off  OutDataTypeStr=boolean
  Logical Operator16 : Logic  AllPortsSameDT=off  OutDataTypeStr=boolean
  Logical Operator2 : Logic  Inputs=4  AllPortsSameDT=off  OutDataTypeStr=boolean
  Logical Operator20 : Logic  Operator=NOT  AllPortsSameDT=off  OutDataTypeStr=boolean
  Logical Operator22 : Logic  AllPortsSameDT=off  OutDataTypeStr=boolean
  Logical Operator3 : Logic  Inputs=4  AllPortsSameDT=off  OutDataTypeStr=boolean
  NOT1 : Logic  Operator=NOT  AllPortsSameDT=off  OutDataTypeStr=boolean
  Relational Operator1 : RelationalOperator  Operator=>  OutDataTypeStr=boolean  RndMeth=Simplest
  Switch1 : Switch  Criteria=u2 ~= 0
  Switch3 : Switch  Criteria=u2 ~= 0
  Switch9 : Switch  Criteria=u2 ~= 0
  Terminator : Terminator
  Test Detection Criteria1 : hcu_lib/Basic_Blocks/Test Detection Criteria
  Timer2 : hcu_lib/Basic_Blocks/Timer
  Unit Delay1 : UnitDelay  SampleTime=-1  HasFrameUpgradeWarning=on
  VDDM_C3BMS1CSDTC_raw32 : Outport
  VDDM_C3BMS1CSCFS_flg : Outport  Port=2
  wires:
  VPMM_HWResetSta_enum/1 -> [VPMM_HWResetSta_enum]
  Logical Operator3/1 -> Switch1/2
  [VDDM_C3BMS1CSChk_flg] -> Switch1/1
  [VPMM_PwrStaSW_enum] -> Equal3/1
  Constant3/1 -> Equal3/2
  [VDDM_C3BMS1LCCFS_flg] -> Logical Operator1/1
  Constant5/1 -> Equal4/2
  [VPMM_HWResetSta_enum] -> Equal4/1
  Equal4/1 -> Logical Operator3/4
  Equal3/1 -> Logical Operator3/2
  Constant4/1 -> Switch1/3
  [No_CAN3_BUS_OFF] -> Logical Operator3/1
  Logical Operator1/1 -> Logical Operator3/3
  [VPMM_HWResetSta_enum] -> Equal2/1
  Equal2/1 -> Logical Operator2/4
  Constant2/1 -> Equal2/2
  Logical Operator2/1 -> Switch3/2
  [VDDM_C3BMS1CSCFS_flg] -> VDDM_C3BMS1CSCFS_flg/1
  [task_time_s] -> Timer2/3
  Timer2/1 -> Equal6/1
  [VDDM_C3BMS1LCCFS_flg] -> Logical Operator10/1
  [VDDM_C3BMS1CSChk_flg] -> Switch3/1
  Logical Operator20/1 -> Timer2/1
  Logical Operator16/1 -> Logical Operator14/1
  Relational Operator1/1 -> Terminator/1  "VDDM_C3BMS1CSDFS_flg"
  Constant1/1 -> DTC_Couter1/3
  Test Detection Criteria1/1 -> [VDDM_C3BMS1CSDet_flg]  "VDDM_C3BMS1CSDet_flg"
  Constant12/1 -> Equal1/2
  [VDDM_C3BMS1CSCFS_flg] -> Delay1/1
  Equal7/1 -> Logical Operator16/1
  Equal6/1 -> [VDDM_C3BMS1CSPass_flg]  "VDDM_C3BMS1CSPass_flg"
  [VPMM_PowerSta_enum] -> Unit Delay1/1
  [VDDM_C3BMS1CSDet_flg] -> DTC_Couter1/1
  DTC_Couter1/1 -> [VDDM_C3BMS1CSCFS_flg]  "VDDM_C3BMS1CSCFS_flg"
  [VPMM_PwrStaSW_enum] -> Equal1/1
  Constant31/1 -> Equal7/2
  [VDDM_C3BMS1CSPass_flg] -> Logical Operator22/1
  Constant33/1 -> Test Detection Criteria1/4
  Constant32/1 -> Test Detection Criteria1/3
  Unit Delay1/1 -> Equal7/1
  Switch1/1 -> Logical Operator20/1, Timer2/2
  Equal1/1 -> Logical Operator2/2
  [DTC_clear_request] -> Logical Operator14/2
  Constant14/1 -> Timer2/4
  [VDDM_C3BMS1CSCFSRls_flg] -> DTC_Couter1/2
  Delay1/1 -> NOT1/1
  DTC_Couter1/2 -> Relational Operator1/1  "VDDM_C3BMS1CSDTC_cnt"
  Constant11/1 -> Relational Operator1/2
  Constant13/1 -> Switch3/3
  Logical Operator10/1 -> Logical Operator2/3
  Constant10/1 -> Equal8/2
  Constant9/1 -> Switch9/1
  [No_CAN3_BUS_OFF] -> Logical Operator2/1
  Switch3/1 -> Switch9/3
  [task_time_s] -> Test Detection Criteria1/2
  [VPMM_PowerSta_enum] -> Equal8/1
  Equal8/1 -> Logical Operator16/2
  NOT1/1 -> Logical Operator22/2
  Logical Operator22/1 -> Logical Operator14/3
  Constant30/1 -> Logical Operator14/4
  Switch9/1 -> Test Detection Criteria1/1
  Logical Operator14/1 -> [VDDM_C3BMS1CSCFSRls_flg]  "VDDM_C3BMS1CSCFSRls_flg"
  Constant7/1 -> Equal6/2
  [VDDM_C3BMS1CSCFSRls_flg] -> Switch9/2
  task_time_s/1 -> [task_time_s]
  VDDM_C3BMS1CSChk_flg/1 -> [VDDM_C3BMS1CSChk_flg]
  VPMM_PwrStaSW_enum/1 -> [VPMM_PwrStaSW_enum]
  VPMM_PowerSta_enum/1 -> [VPMM_PowerSta_enum]
  VDDM_C3BMS1LCCFS_flg/1 -> [VDDM_C3BMS1LCCFS_flg]
  No_CAN3_BUS_OFF/1 -> [No_CAN3_BUS_OFF]
  DTC_clear_request/1 -> [DTC_clear_request]
  DTC_Info/1 -> VDDM_C3BMS1CSDTC_raw32/1  "VDDM_C3BMS1CSDTC_raw32"
  [VDDM_C3BMS1CSCFS_flg] -> DTC_Info/3
  [VDDM_C3BMS1CSDet_flg] -> DTC_Info/1
  [VDDM_C3BMS1CSPass_flg] -> DTC_Info/2
  [DTC_clear_request] -> DTC_Info/4

== system ddm/DDM/DDM/PMM/Comm err/The CAN signal between VCU and BMS6 is discontinuous1 ==
  note: Test Detection Criteria
  note: Test Pass Criteria
  note: Release Condition After Decision
  note: Diagnostics and Fault Handling
  task_time_s : Inport
  VPMM_PowerSta_enum : Inport  Port=2
  VPMM_PwrStaSW_enum : Inport  Port=3
  VDDM_C3BMS6RCChk_flg : Inport  Port=4
  VDDM_C3BMS6LCCFS_flg : Inport  Port=5
  No_CAN3_BUS_OFF : Inport  Port=6
  DTC_clear_request : Inport  Port=7
  VPMM_HWResetSta_enum : Inport  Port=8
  Constant1 : Constant  Value=ENUM_HWRESETSTA_HWRESETING
  Constant10 : Constant  Value=ENUM_POWERSTA_STANDBY
  Constant11 : Constant  Value=ZERO_INT
  Constant18 : Constant  Value=KDDM_C3BMS6RCPassTO_s
  Constant19 : Constant  Value=KDDM_C3BMS6RCPassTO_s
  Constant2 : Constant  Value=FALSE
  Constant3 : Constant  Value=ENUM_PWRSTASW_OFF
  Constant4 : Constant  Value=FALSE
  Constant40 : Constant  Value=KDDM_C3BMS6RCDTC_cnt
  Constant41 : Constant  Value=KDDM_C3BMS6RCDetTO_s
  Constant48 : Constant  Value=KDDM_C3BMS6RCDTC_cnt
  Constant5 : Constant  Value=ENUM_HWRESETSTA_HWRESETING
  Constant6 : Constant  Value=ENUM_PWRSTASW_OFF
  Constant7 : Constant  Value=KDDM_CommErrDiagnosisOffSW_flg
  Constant8 : Constant  Value=ENUM_POWERSTA_OFF
  Constant9 : Constant  Value=TRUE
  DTC_Couter : hcu_lib/Basic_Blocks/DTC_Couter
  DTC_Info : hcu_lib/Basic_Blocks/DTC_Info
  Delay1 : Delay  DelayLength=1
  Equal{,1..2,5} (4 alike) : RelationalOperator  Operator=~=  OutDataTypeStr=boolean  RndMeth=Simplest
  Equal3 : RelationalOperator  OutDataTypeStr=boolean  RndMeth=Simplest
  Equal4 : RelationalOperator  Operator===  OutDataTypeStr=boolean  RndMeth=Simplest
  Equal6 : RelationalOperator  Operator===  OutDataTypeStr=boolean  RndMeth=Simplest
  Logical Operator1 : Logic  Operator=NOT  AllPortsSameDT=off  OutDataTypeStr=boolean
  Logical Operator14 : Logic  Operator=OR  Inputs=4  AllPortsSameDT=off  OutDataTypeStr=boolean
  Logical Operator16 : Logic  AllPortsSameDT=off  OutDataTypeStr=boolean
  Logical Operator2 : Logic  Inputs=4  AllPortsSameDT=off  OutDataTypeStr=boolean
  Logical Operator3 : Logic  Operator=NOT  AllPortsSameDT=off  OutDataTypeStr=boolean
  Logical Operator4 : Logic  Inputs=4  AllPortsSameDT=off  OutDataTypeStr=boolean
  Logical Operator6 : Logic  Operator=NOT  AllPortsSameDT=off  OutDataTypeStr=boolean
  Logical Operator8 : Logic  AllPortsSameDT=off  OutDataTypeStr=boolean
  NOT1 : Logic  Operator=NOT  AllPortsSameDT=off  OutDataTypeStr=boolean
  Relational Operator1 : RelationalOperator  Operator=>  OutDataTypeStr=boolean  RndMeth=Simplest
  Switch1 : Switch  Criteria=u2 ~= 0
  Switch3 : Switch  Criteria=u2 ~= 0
  Switch6 : Switch  Criteria=u2 ~= 0
  Terminator : Terminator
  Test Detection Criteria : hcu_lib/Basic_Blocks/Test Detection Criteria
  Timer1 : hcu_lib/Basic_Blocks/Timer
  Unit Delay1 : UnitDelay  SampleTime=-1  HasFrameUpgradeWarning=on
  VDDM_C3BMS6RCDTC_raw32 : Outport
  VDDM_C3BMS6RCCFS_flg : Outport  Port=2
  wires:
  [VPMM_PwrStaSW_enum] -> Equal1/1
  [No_CAN3_BUS_OFF] -> Logical Operator4/1
  Constant6/1 -> Equal1/2
  Equal2/1 -> Logical Operator4/4
  Constant9/1 -> Switch1/3
  [VDDM_C3BMS6LCCFS_flg] -> Logical Operator3/1
  [VDDM_C3BMS6RCChk_flg] -> Switch1/1
  Equal1/1 -> Logical Operator4/2
  Logical Operator3/1 -> Logical Operator4/3
  Logical Operator4/1 -> Switch1/2
  [VPMM_HWResetSta_enum] -> Equal2/1
  Constant5/1 -> Equal2/2
  Equal5/1 -> Logical Operator2/4
  Constant1/1 -> Equal5/2
  [VPMM_HWResetSta_enum] -> Equal5/1
  VPMM_HWResetSta_enum/1 -> [VPMM_HWResetSta_enum]
  Relational Operator1/1 -> Terminator/1  "VDDM_C3BMS6RCDFS_flg"
  Constant11/1 -> Relational Operator1/2
  [VDDM_C3BMS6RCCFSRls_flg] -> DTC_Couter/2
  Delay1/1 -> NOT1/1
  [VDDM_C3BMS6RCPass_flg] -> Logical Operator8/1
  Equal6/1 -> Logical Operator16/2
  Logical Operator8/1 -> Logical Operator14/3
  Logical Operator14/1 -> [VDDM_C3BMS6RCCFSRls_flg]  "VDDM_C3BMS6RCCFSRls_flg"
  Constant10/1 -> Equal6/2
  [VDDM_C3BMS6RCCFS_flg] -> Delay1/1
  NOT1/1 -> Logical Operator8/2
  Constant7/1 -> Logical Operator14/4
  [VPMM_PowerSta_enum] -> Unit Delay1/1
  Constant8/1 -> Equal4/2
  Equal4/1 -> Logical Operator16/1
  Logical Operator16/1 -> Logical Operator14/1
  [VPMM_PowerSta_enum] -> Equal6/1
  Unit Delay1/1 -> Equal4/1
  [DTC_clear_request] -> Logical Operator14/2
  task_time_s/1 -> [task_time_s]
  VDDM_C3BMS6RCChk_flg/1 -> [VDDM_C3BMS6RCChk_flg]
  VPMM_PwrStaSW_enum/1 -> [VPMM_PwrStaSW_enum]
  VPMM_PowerSta_enum/1 -> [VPMM_PowerSta_enum]
  No_CAN3_BUS_OFF/1 -> [No_CAN3_BUS_OFF]
  Logical Operator2/1 -> Switch3/2
  [task_time_s] -> Test Detection Criteria/2
  Constant40/1 -> Test Detection Criteria/3
  Switch3/1 -> Switch6/3
  Constant3/1 -> Equal/2
  Constant4/1 -> Switch3/3
  [VDDM_C3BMS6RCChk_flg] -> Switch3/1
  Equal/1 -> Logical Operator2/2
  [No_CAN3_BUS_OFF] -> Logical Operator2/1
  Equal3/1 -> [VDDM_C3BMS6RCPass_flg]  "VDDM_C3BMS6RCPass_flg"
  Logical Operator6/1 -> Timer1/1
  Constant19/1 -> Equal3/2
  Switch1/1 -> Logical Operator6/1, Timer1/2
  Timer1/1 -> Equal3/1
  Constant18/1 -> Timer1/4
  DTC_clear_request/1 -> [DTC_clear_request]
  VDDM_C3BMS6LCCFS_flg/1 -> [VDDM_C3BMS6LCCFS_flg]
  [VDDM_C3BMS6LCCFS_flg] -> Logical Operator1/1
  Logical Operator1/1 -> Logical Operator2/3
  [VPMM_PwrStaSW_enum] -> Equal/1
  [task_time_s] -> Timer1/3
  [VDDM_C3BMS6RCCFS_flg] -> DTC_Info/3
  DTC_Info/1 -> VDDM_C3BMS6RCDTC_raw32/1  "VDDM_C3BMS6RCDTC_raw32"
  Test Detection Criteria/1 -> [VDDM_C3BMS6RCDet_flg]  "VDDM_C3BMS6RCDet_flg"
  Constant41/1 -> Test Detection Criteria/4
  [VDDM_C3BMS6RCDet_flg] -> DTC_Info/1
  [VDDM_C3BMS6RCPass_flg] -> DTC_Info/2
  [DTC_clear_request] -> DTC_Info/4
  Constant2/1 -> Switch6/1
  Switch6/1 -> Test Detection Criteria/1
  [VDDM_C3BMS6RCCFSRls_flg] -> Switch6/2
  [VDDM_C3BMS6RCCFS_flg] -> VDDM_C3BMS6RCCFS_flg/1
  Constant48/1 -> DTC_Couter/3
  DTC_Couter/1 -> [VDDM_C3BMS6RCCFS_flg]  "VDDM_C3BMS6RCCFS_flg"
  [VDDM_C3BMS6RCDet_flg] -> DTC_Couter/1
  DTC_Couter/2 -> Relational Operator1/1  "VDDM_C3BMS6RCDTC_cnt"

== system ddm/DDM/DDM/PMM/Comm err/The CAN signal between VCU and BMS6 is incomplete1 ==
  note: Test Detection Criteria
  note: Test Pass Criteria
  note: Release Condition After Decision
  note: Diagnostics and Fault Handling
  task_time_s : Inport
  VPMM_PowerSta_enum : Inport  Port=2
  VPMM_PwrStaSW_enum : Inport  Port=3
  VDDM_C3BMS6CSChk_flg : Inport  Port=4
  VDDM_C3BMS6LCCFS_flg : Inport  Port=5
  No_CAN3_BUS_OFF : Inport  Port=6
  DTC_clear_request : Inport  Port=7
  VPMM_HWResetSta_enum : Inport  Port=8
  Constant1 : Constant  Value=ENUM_HWRESETSTA_HWRESETING
  Constant10 : Constant  Value=ENUM_POWERSTA_STANDBY
  Constant11 : Constant  Value=ZERO_INT
  Constant12 : Constant  Value=ENUM_PWRSTASW_OFF
  Constant13 : Constant  Value=FALSE
  Constant14 : Constant  Value=KDDM_C3BMS6CSPassTO_s
  Constant2 : Constant  Value=ENUM_HWRESETSTA_HWRESETING
  Constant27 : Constant  Value=KDDM_C3BMS6CSDTC_cnt
  Constant3 : Constant  Value=ENUM_PWRSTASW_OFF
  Constant30 : Constant  Value=KDDM_CommErrDiagnosisOffSW_flg
  Constant31 : Constant  Value=ENUM_POWERSTA_OFF
  Constant32 : Constant  Value=KDDM_C3BMS6CSDTC_cnt
  Constant33 : Constant  Value=KDDM_C3BMS6CSDetTO_s
  Constant4 : Constant  Value=TRUE
  Constant7 : Constant  Value=KDDM_C3BMS6CSPassTO_s
  Constant9 : Constant  Value=FALSE
  DTC_Couter1 : hcu_lib/Basic_Blocks/DTC_Couter
  DTC_Info : hcu_lib/Basic_Blocks/DTC_Info
  Delay1 : Delay  DelayLength=1
  Equal{1..4} (4 alike) : RelationalOperator  Operator=~=  OutDataTypeStr=boolean  RndMeth=Simplest
  Equal6 : RelationalOperator  OutDataTypeStr=boolean  RndMeth=Simplest
  Equal7 : RelationalOperator  Operator===  OutDataTypeStr=boolean  RndMeth=Simplest
  Equal8 : RelationalOperator  Operator===  OutDataTypeStr=boolean  RndMeth=Simplest
  Logical Operator1 : Logic  Operator=NOT  AllPortsSameDT=off  OutDataTypeStr=boolean
  Logical Operator10 : Logic  Operator=NOT  AllPortsSameDT=off  OutDataTypeStr=boolean
  Logical Operator14 : Logic  Operator=OR  Inputs=4  AllPortsSameDT=off  OutDataTypeStr=boolean
  Logical Operator16 : Logic  AllPortsSameDT=off  OutDataTypeStr=boolean
  Logical Operator2 : Logic  Inputs=4  AllPortsSameDT=off  OutDataTypeStr=boolean
  Logical Operator20 : Logic  Operator=NOT  AllPortsSameDT=off  OutDataTypeStr=boolean
  Logical Operator22 : Logic  AllPortsSameDT=off  OutDataTypeStr=boolean
  Logical Operator3 : Logic  Inputs=4  AllPortsSameDT=off  OutDataTypeStr=boolean
  NOT1 : Logic  Operator=NOT  AllPortsSameDT=off  OutDataTypeStr=boolean
  Relational Operator1 : RelationalOperator  Operator=>  OutDataTypeStr=boolean  RndMeth=Simplest
  Switch1 : Switch  Criteria=u2 ~= 0
  Switch3 : Switch  Criteria=u2 ~= 0
  Switch9 : Switch  Criteria=u2 ~= 0
  Terminator : Terminator
  Test Detection Criteria1 : hcu_lib/Basic_Blocks/Test Detection Criteria
  Timer2 : hcu_lib/Basic_Blocks/Timer
  Unit Delay1 : UnitDelay  SampleTime=-1  HasFrameUpgradeWarning=on
  VDDM_C3BMS6CSDTC_raw32 : Outport
  VDDM_C3BMS6CSCFS_flg : Outport  Port=2
  wires:
  VPMM_HWResetSta_enum/1 -> [VPMM_HWResetSta_enum]
  [VPMM_HWResetSta_enum] -> Equal3/1
  Equal4/1 -> Logical Operator3/2
  [No_CAN3_BUS_OFF] -> Logical Operator3/1
  Constant3/1 -> Equal4/2
  [VDDM_C3BMS6LCCFS_flg] -> Logical Operator1/1
  [VPMM_PwrStaSW_enum] -> Equal4/1
  Constant4/1 -> Switch1/3
  Equal3/1 -> Logical Operator3/4
  Constant2/1 -> Equal3/2
  Logical Operator1/1 -> Logical Operator3/3
  [VDDM_C3BMS6CSChk_flg] -> Switch1/1
  Logical Operator3/1 -> Switch1/2
  Constant1/1 -> Equal1/2
  [VPMM_HWResetSta_enum] -> Equal1/1
  Equal1/1 -> Logical Operator2/4
  Test Detection Criteria1/1 -> [VDDM_C3BMS6CSDet_flg]  "VDDM_C3BMS6CSDet_flg"
  DTC_Couter1/2 -> Relational Operator1/1  "VDDM_C3BMS6CSDTC_cnt"
  Constant14/1 -> Timer2/4
  DTC_Couter1/1 -> [VDDM_C3BMS6CSCFS_flg]  "VDDM_C3BMS6CSCFS_flg"
  Delay1/1 -> NOT1/1
  [VDDM_C3BMS6CSDet_flg] -> DTC_Couter1/1
  Logical Operator16/1 -> Logical Operator14/1
  Unit Delay1/1 -> Equal7/1
  Equal2/1 -> Logical Operator2/2
  [DTC_clear_request] -> Logical Operator14/2
  Constant31/1 -> Equal7/2
  Equal7/1 -> Logical Operator16/1
  [VPMM_PowerSta_enum] -> Equal8/1
  Switch9/1 -> Test Detection Criteria1/1
  Constant30/1 -> Logical Operator14/4
  Constant10/1 -> Equal8/2
  [task_time_s] -> Timer2/3
  Logical Operator14/1 -> [VDDM_C3BMS6CSCFSRls_flg]  "VDDM_C3BMS6CSCFSRls_flg"
  [VDDM_C3BMS6CSCFS_flg] -> Delay1/1
  Constant32/1 -> Test Detection Criteria1/3
  [VPMM_PowerSta_enum] -> Unit Delay1/1
  Relational Operator1/1 -> Terminator/1  "VDDM_C3BMS6CSDFS_flg"
  NOT1/1 -> Logical Operator22/2
  Logical Operator22/1 -> Logical Operator14/3
  Equal8/1 -> Logical Operator16/2
  Constant12/1 -> Equal2/2
  [VDDM_C3BMS6CSPass_flg] -> Logical Operator22/1
  [task_time_s] -> Test Detection Criteria1/2
  Switch3/1 -> Switch9/3
  Logical Operator2/1 -> Switch3/2
  [No_CAN3_BUS_OFF] -> Logical Operator2/1
  Constant27/1 -> DTC_Couter1/3
  [VDDM_C3BMS6CSChk_flg] -> Switch3/1
  Equal6/1 -> [VDDM_C3BMS6CSPass_flg]  "VDDM_C3BMS6CSPass_flg"
  [VDDM_C3BMS6CSCFSRls_flg] -> Switch9/2
  [VPMM_PwrStaSW_enum] -> Equal2/1
  Constant9/1 -> Switch9/1
  Constant33/1 -> Test Detection Criteria1/4
  Logical Operator10/1 -> Logical Operator2/3
  Constant7/1 -> Equal6/2
  [VDDM_C3BMS6LCCFS_flg] -> Logical Operator10/1
  Switch1/1 -> Logical Operator20/1, Timer2/2
  Timer2/1 -> Equal6/1
  Constant13/1 -> Switch3/3
  Logical Operator20/1 -> Timer2/1
  [VDDM_C3BMS6CSCFSRls_flg] -> DTC_Couter1/2
  Constant11/1 -> Relational Operator1/2
  No_CAN3_BUS_OFF/1 -> [No_CAN3_BUS_OFF]
  VPMM_PowerSta_enum/1 -> [VPMM_PowerSta_enum]
  VPMM_PwrStaSW_enum/1 -> [VPMM_PwrStaSW_enum]
  VDDM_C3BMS6CSChk_flg/1 -> [VDDM_C3BMS6CSChk_flg]
  task_time_s/1 -> [task_time_s]
  DTC_clear_request/1 -> [DTC_clear_request]
  VDDM_C3BMS6LCCFS_flg/1 -> [VDDM_C3BMS6LCCFS_flg]
  [VDDM_C3BMS6CSPass_flg] -> DTC_Info/2
  [VDDM_C3BMS6CSCFS_flg] -> DTC_Info/3
  DTC_Info/1 -> VDDM_C3BMS6CSDTC_raw32/1  "VDDM_C3BMS6CSDTC_raw32"
  [VDDM_C3BMS6CSDet_flg] -> DTC_Info/1
  [DTC_clear_request] -> DTC_Info/4
  [VDDM_C3BMS6CSCFS_flg] -> VDDM_C3BMS6CSCFS_flg/1
